simulink model "three_tank_linearization"  (R2020b)
settings: Solver=ode15s  StartTime=0.0  StopTime=2000  FixedStep=1  RelTol=1e-8  EnableMultiTasking=on
libraries: simulink x7, pid_lib x3
settings Model: Creator=Karl  LastModifiedBy=Fuzz4
settings SolverCC: AlgebraicLoopSolver=LineSearch  AutoInsertRateTranBlk=on
settings DataIOCC: SaveFormat=Array  ReturnWorkspaceOutputs=off  OutputOption=SpecifiedOutputTimes  OutputTimes=[0:2000]
settings OptimizationCC: LifeSpan=inf
settings DebuggingCC: AlgebraicLoopMsg=none  UnderspecifiedInitializationDetection=Classic  MergeDetectMultiDrivingBlocksExec=none  SFUnexpectedBacktrackingDiag=warning  SFNoUnconditionalDefaultTransitionDiag=warning  SFExecutionAtInitializationDiag=none  ArithmeticOperatorsInVariantConditions=warning
settings HardwareCC: ProdBitPerPointer=32  ProdBitPerSizeT=32  ProdBitPerPtrDiffT=32  ProdLargestAtomicFloat=None  ProdIntDivRoundTo=Undefined  ProdEndianess=Unspecified  ProdWordSize=32  ProdHWDeviceType=32-bit Generic
settings ModelReferenceCC: PropagateSignalLabelsOutOfModel=off
settings SFSimCC: SimUseLocalCustomCode=off  CustomCodeUndefinedFunction=UseInterfaceOnly
settings RTWCC: RTWUseLocalCustomCode=off
settings CodeAppCC: StateflowObjectComments=on
settings GRTTargetCC: TargetLangStandard=C89/C90 (ANSI)
settings ConfigComp: CovMetricSettings=dw  CovSaveCumulativeToWorkspaceVar=on  CovSaveSingleToWorkspaceVar=on  CovExternalEMLEnable=off

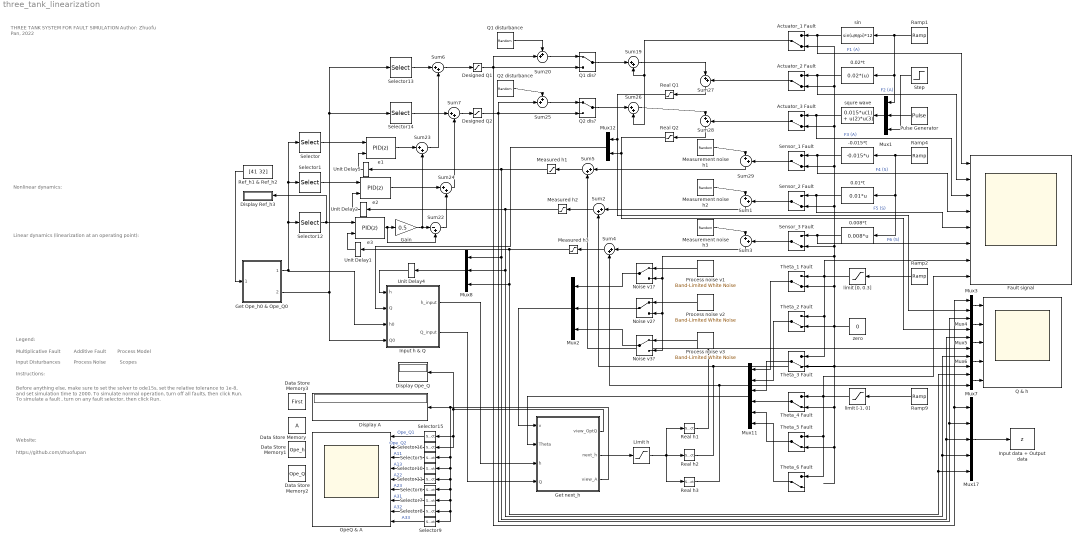
== system three_tank_linearization ==
  note: THREE TANK SYSTEM
      | FOR FAULT SIMULATION
      |
      | Author: Zhuofu Pan, 2022
  note: Multiplicative Fault
  note: Process Noise
  note: Process Model
  note: Input Disturbances
  note: Scopes
  note: Nonlinear dynamics:
  note: Linear dynamics
      | (linearization at an operating point):
  note: Before anything else, make sure to set the solver to ode15s, set the relative tolerance to 1e-8, and set simulation time to 2000.
      |
      | To simulate normal operation, turn off all faults, then click Run.
      |
      | To simulate a fault , turn on any fault selector, then click Run.
  note: Legend:
  note: Instructions:
  note: Website:
  note: https://github.com/zhuofupan
  note: Additive Fault
  " zero" : Constant  Value=0
  -0.015*t : Fcn  Expr=-0.015*u
  0.008*t : Fcn  Expr=0.008*u
  0.01*t : Fcn  Expr=0.01*u
  0.02*t : Fcn  Expr=0.02*(u)
  Actuator_1 Fault : ManualSwitch  CurrentSetting=0
  Actuator_2 Fault : ManualSwitch  CurrentSetting=0
  Actuator_3 Fault : ManualSwitch  CurrentSetting=0
  Data Store Memory : DataStoreMemory  ReadBeforeWriteMsg=warning  WriteAfterWriteMsg=warning  WriteAfterReadMsg=warning  ShowAdditionalParam=off  OutDataTypeStr=double  Dimensions=[3,3]
  Data Store Memory1 : DataStoreMemory  DataStoreName=Ope_h  ReadBeforeWriteMsg=warning  WriteAfterWriteMsg=warning  WriteAfterReadMsg=warning  ShowAdditionalParam=off  OutMin=0  OutMax=62  OutDataTypeStr=double  Dimensions=3
  Data Store Memory2 : DataStoreMemory  DataStoreName=Ope_Q  ReadBeforeWriteMsg=warning  WriteAfterWriteMsg=warning  WriteAfterReadMsg=warning  ShowAdditionalParam=off  OutMin=0  OutMax=150  OutDataTypeStr=double  Dimensions=2
  Data Store Memory3 : DataStoreMemory  DataStoreName=First  ReadBeforeWriteMsg=warning  WriteAfterWriteMsg=warning  WriteAfterReadMsg=warning  InitialValue=true  ShowAdditionalParam=off  OutDataTypeStr=boolean  Dimensions=1
  Designed Q1 : Saturate  UpperLimit=150  LowerLimit=0
  Designed Q2 : Saturate  UpperLimit=150  LowerLimit=0
  Display A : Display
      settings: Decimation=2
  Display Ope_Q : Display
  Display Ref_h3 : Display
  Fault signal : Scope  NumInputPorts=8
  Gain : Gain  Gain=0.5
  Get Ope_h0 & Ope_Q0 : MATLAB Function  TreatAsAtomicUnit=on
  Get next_h : MATLAB Function  TreatAsAtomicUnit=on
  Input data + Output data : ToWorkspace  VariableName=z  SampleTime=-1
  Input h & Q : MATLAB Function  TreatAsAtomicUnit=on
      settings: RTWSystemCode=Nonreusable function
  Limit h : Saturate  UpperLimit=62  LowerLimit=0
  Measured h1 : Saturate  UpperLimit=62  LowerLimit=0
  Measured h2 : Saturate  UpperLimit=62  LowerLimit=0
  Measured h3 : Saturate  UpperLimit=62  LowerLimit=0
  Measurement noise h1 : RandomNumber  Variance=0.01  Seed=randi(100000)
  Measurement noise h2 : RandomNumber  Variance=0.01  Seed=randi(100000)
  Measurement noise h3 : RandomNumber  Variance=0.01  Seed=randi(100000)
  Mux1 : Mux  Inputs=3
  Mux11 : Mux  Inputs=6
  Mux{3..7,12} (6 alike) : Mux  Inputs=2
  Mux17 : Mux  Inputs=5
  Mux2 : Mux  Inputs=3
  Mux8 : Mux  Inputs=3
  Noise v1? : ManualSwitch
  Noise v2? : ManualSwitch
  Noise v3? : ManualSwitch
  OpeQ & A : Scope  NumInputPorts=9
  Process noise v1 : simulink/Sources/Band-Limited White Noise  Cov=[1e-4]  Ts=1  seed=randi(100000)
  Process noise v2 : simulink/Sources/Band-Limited White Noise  Cov=[1e-4]  Ts=1  seed=randi(100000)
  Process noise v3 : simulink/Sources/Band-Limited White Noise  Cov=[1e-4]  Ts=1  seed=randi(100000)
  Pulse Generator : DiscretePulseGenerator  PulseType=Time based  Amplitude=5  Period=120  PulseWidth=80
  Q & h : Scope  NumInputPorts=5
  Q1 dis? : ManualSwitch
  Q1 disturbance : RandomNumber  Variance=0.01  Seed=randi(100000)  SampleTime=15
  Q2 dis? : ManualSwitch
  Q2 disturbance : RandomNumber  Variance=0.01  Seed=randi(100000)  SampleTime=15
  Ramp1 : simulink/Sources/Ramp  slope=1  start=200  InitialOutput=0
  Ramp2 : simulink/Sources/Ramp  slope=0.00005  start=200  InitialOutput=0
  Ramp4 : simulink/Sources/Ramp  slope=1  start=200  InitialOutput=0
  Ramp9 : simulink/Sources/Ramp  slope=-0.001  start=200  InitialOutput=0
  Real Q1 : Saturate  UpperLimit=150  LowerLimit=0
  Real Q2 : Saturate  UpperLimit=150  LowerLimit=0
  Real h1 : Selector  InputPortWidth=3  IndexOptions=Index vector (dialog)  Indices=1  OutputSizes=1
  Real h2 : Selector  InputPortWidth=3  IndexOptions=Index vector (dialog)  Indices=2  OutputSizes=1
  Real h3 : Selector  InputPortWidth=3  IndexOptions=Index vector (dialog)  Indices=3  OutputSizes=1
  Ref_h1 & Ref_h2 : Constant  Value=[41 32]
  Selector : Selector  InputPortWidth=3  IndexOptions=Index vector (dialog)  Indices=1  OutputSizes=1
  Selector1 : Selector  InputPortWidth=3  IndexOptions=Index vector (dialog)  Indices=2  OutputSizes=1
  Selector10 : Selector  NumberOfDimensions=2  InputPortWidth=2  IndexOptions=Index vector (dialog),Index vector (dialog)  Indices=1,3  OutputSizes=1,1
  Selector11 : Selector  NumberOfDimensions=2  InputPortWidth=2  IndexOptions=Index vector (dialog),Index vector (dialog)  Indices=2,2  OutputSizes=1,1
  Selector12 : Selector  InputPortWidth=3  IndexOptions=Index vector (dialog)  Indices=3  OutputSizes=1
  Selector13 : Selector  InputPortWidth=2  IndexOptions=Index vector (dialog)  Indices=1  OutputSizes=1
  Selector14 : Selector  InputPortWidth=2  IndexOptions=Index vector (dialog)  Indices=2  OutputSizes=1
  Selector15 : Selector  InputPortWidth=2  IndexOptions=Index vector (dialog)  Indices=1  OutputSizes=1
  Selector16 : Selector  InputPortWidth=2  IndexOptions=Index vector (dialog)  Indices=2  OutputSizes=1
  Selector5 : Selector  NumberOfDimensions=2  InputPortWidth=2  IndexOptions=Index vector (dialog),Index vector (dialog)  Indices=1,1  OutputSizes=1,1
  Selector6 : Selector  NumberOfDimensions=2  InputPortWidth=2  IndexOptions=Index vector (dialog),Index vector (dialog)  Indices=2,3  OutputSizes=1,1
  Selector7 : Selector  NumberOfDimensions=2  InputPortWidth=2  IndexOptions=Index vector (dialog),Index vector (dialog)  Indices=3,1  OutputSizes=1,1
  Selector8 : Selector  NumberOfDimensions=2  InputPortWidth=2  IndexOptions=Index vector (dialog),Index vector (dialog)  Indices=3,2  OutputSizes=1,1
  Selector9 : Selector  NumberOfDimensions=2  InputPortWidth=2  IndexOptions=Index vector (dialog),Index vector (dialog)  Indices=3,3  OutputSizes=1,1
  Sensor_1 Fault : ManualSwitch  CurrentSetting=0
  Sensor_2 Fault : ManualSwitch  CurrentSetting=0
  Sensor_3 Fault : ManualSwitch  CurrentSetting=0
  Step : Step  Time=200  SampleTime=1
  Sum{1..7,19,23..24,26..29} (14 alike) : Sum  Inputs=|++
  Sum20 : Sum  Inputs=++|
  Sum22 : Sum  Inputs=|-+
  Sum25 : Sum  Inputs=++|
  Theta_1 Fault : ManualSwitch  CurrentSetting=0
  Theta_2 Fault : ManualSwitch  CurrentSetting=0
  Theta_3 Fault : ManualSwitch  CurrentSetting=0
  Theta_4 Fault : ManualSwitch  CurrentSetting=0
  Theta_5 Fault : ManualSwitch  CurrentSetting=0
  Theta_6 Fault : ManualSwitch  CurrentSetting=0
  Unit Delay{1..2,4..5} (4 alike) : UnitDelay  SampleTime=-1  HasFrameUpgradeWarning=on
  e1 : pid_lib/PID Controller (2DOF)  Controller=PID  Form=Parallel  TimeDomain=Discrete-time  UseExternalTs=off  SampleTime=-1  IntegratorMethod=Forward Euler  FilterMethod=Forward Euler  ControllerParametersSource=internal  P=0.02  I=0.02  D=0  UseFilter=on  N=100  b=1  c=1  TunerSelectOption=Transfer Function Based (PID Tuner App)  InitialConditionSource=internal  InitialConditionForIntegrator=0  InitialConditionForFilter=0  DifferentiatorICPrevScaledInput=0  ExternalReset=none  TrackingMode=off  Kt=1  LimitOutput=off  SatLimitsSource=internal  UpperSaturationLimit=inf  LowerSaturationLimit=-inf  LinearizeAsGain=on  AntiWindupMode=none  Kb=1  POutMin=[]  POutMax=[]  IOutMin=[]  IOutMax=[]  DOutMin=[]  DOutMax=[]  NOutMin=[]  NOutMax=[]  bOutMin=[]  bOutMax=[]  cOutMin=[]  cOutMax=[]  SumOutMin=[]  SumOutMax=[]  SaturationOutMin=[]  SaturationOutMax=[]  PParamMin=[]  PParamMax=[]  IParamMin=[]  IParamMax=[]  DParamMin=[]  DParamMax=[]  NParamMin=[]  NParamMax=[]  bParamMin=[]  bParamMax=[]  cParamMin=[]  cParamMax=[]  KbParamMin=[]  KbParamMax=[]  KtParamMin=[]  KtParamMax=[]  KbOutMin=[]  KbOutMax=[]  KtOutMin=[]  KtOutMax=[]  IntegratorOutMin=[]  IntegratorOutMax=[]  FilterOutMin=[]  FilterOutMax=[]  SumI1OutMin=[]  SumI1OutMax=[]  SumI2OutMin=[]  SumI2OutMax=[]  SumI3OutMin=[]  SumI3OutMax=[]  SumI4OutMin=[]  SumI4OutMax=[]  SumDOutMin=[]  SumDOutMax=[]  Sum1OutMin=[]  Sum1OutMax=[]  Sum2OutMin=[]  Sum2OutMax=[]  Sum3OutMin=[]  Sum3OutMax=[]  DifferentiatorOutMin=[]  DifferentiatorOutMax=[]  FilterDiffOutCoefMin=[]  FilterDiffOutCoefMax=[]  ReciprocalOutMin=[]  ReciprocalOutMax=[]  SumDenOutMin=[]  SumDenOutMax=[]  SumNumOutMin=[]  SumNumOutMax=[]  DivideOutMin=[]  DivideOutMax=[]  UdiffTsProdOutMin=[]  UdiffTsProdOutMax=[]  NTsProdOutMin=[]  NTsProdOutMax=[]  UintegralTsProdOutMin=[]  UintegralTsProdOutMax=[]  UngainTsProdOutMin=[]  UngainTsProdOutMax=[]  IntegratorContinuousStateAttributes=''  IntegratorStateMustResolveToSignalObject=off  IntegratorRTWStateStorageClass=Auto  FilterContinuousStateAttributes=''  FilterStateMustResolveToSignalObject=off  FilterRTWStateStorageClass=Auto  ParallelPVariant=InternalParameters  IdealPVariant=Disabled  IVariant=InternalParameters  DVariant=InternalParameters  bVariant=InternalParameters  cVariant=InternalParameters  IntegratorVariant=Discrete  SatVariant=Disabled  AWVariant=Passthrough  PCopyVariant=Disabled  TRVariant=Disabled  FdbkBlocksVariant=Forward  IdealPFdbkVariant=Disabled  SatFdbkVariant=Disabled  DerivativeFilterVariant=ForwardEulerFilter  NVariant=InternalParameters  NCopyVariant=Disabled  FilterICVariant=InternalICsFilter  IntegratorICVariant=InternalICs  ExternalResetVariant=Disabled  TRSumVariant=Passthrough  SumFdbkVariant=Disabled  SumVariant=Sum_PID  TsampFilterVariant=InternalTs  TsampNgainVariant=Passthrough  TsampIntegralVariant=Passthrough  ExternalSaturationOutDataTypeStr=Inherit: Same as second input
      settings: SourceProductBaseCode=SL
  e2 : pid_lib/PID Controller (2DOF)  Controller=PID  Form=Parallel  TimeDomain=Discrete-time  UseExternalTs=off  SampleTime=-1  IntegratorMethod=Forward Euler  FilterMethod=Forward Euler  ControllerParametersSource=internal  P=0.02  I=0.02  D=0  UseFilter=on  N=100  b=1  c=1  TunerSelectOption=Transfer Function Based (PID Tuner App)  InitialConditionSource=internal  InitialConditionForIntegrator=0  InitialConditionForFilter=0  DifferentiatorICPrevScaledInput=0  ExternalReset=none  TrackingMode=off  Kt=1  LimitOutput=off  SatLimitsSource=internal  UpperSaturationLimit=inf  LowerSaturationLimit=-inf  LinearizeAsGain=on  AntiWindupMode=none  Kb=1  POutMin=[]  POutMax=[]  IOutMin=[]  IOutMax=[]  DOutMin=[]  DOutMax=[]  NOutMin=[]  NOutMax=[]  bOutMin=[]  bOutMax=[]  cOutMin=[]  cOutMax=[]  SumOutMin=[]  SumOutMax=[]  SaturationOutMin=[]  SaturationOutMax=[]  PParamMin=[]  PParamMax=[]  IParamMin=[]  IParamMax=[]  DParamMin=[]  DParamMax=[]  NParamMin=[]  NParamMax=[]  bParamMin=[]  bParamMax=[]  cParamMin=[]  cParamMax=[]  KbParamMin=[]  KbParamMax=[]  KtParamMin=[]  KtParamMax=[]  KbOutMin=[]  KbOutMax=[]  KtOutMin=[]  KtOutMax=[]  IntegratorOutMin=[]  IntegratorOutMax=[]  FilterOutMin=[]  FilterOutMax=[]  SumI1OutMin=[]  SumI1OutMax=[]  SumI2OutMin=[]  SumI2OutMax=[]  SumI3OutMin=[]  SumI3OutMax=[]  SumI4OutMin=[]  SumI4OutMax=[]  SumDOutMin=[]  SumDOutMax=[]  Sum1OutMin=[]  Sum1OutMax=[]  Sum2OutMin=[]  Sum2OutMax=[]  Sum3OutMin=[]  Sum3OutMax=[]  DifferentiatorOutMin=[]  DifferentiatorOutMax=[]  FilterDiffOutCoefMin=[]  FilterDiffOutCoefMax=[]  ReciprocalOutMin=[]  ReciprocalOutMax=[]  SumDenOutMin=[]  SumDenOutMax=[]  SumNumOutMin=[]  SumNumOutMax=[]  DivideOutMin=[]  DivideOutMax=[]  UdiffTsProdOutMin=[]  UdiffTsProdOutMax=[]  NTsProdOutMin=[]  NTsProdOutMax=[]  UintegralTsProdOutMin=[]  UintegralTsProdOutMax=[]  UngainTsProdOutMin=[]  UngainTsProdOutMax=[]  IntegratorContinuousStateAttributes=''  IntegratorStateMustResolveToSignalObject=off  IntegratorRTWStateStorageClass=Auto  FilterContinuousStateAttributes=''  FilterStateMustResolveToSignalObject=off  FilterRTWStateStorageClass=Auto  ParallelPVariant=InternalParameters  IdealPVariant=Disabled  IVariant=InternalParameters  DVariant=InternalParameters  bVariant=InternalParameters  cVariant=InternalParameters  IntegratorVariant=Discrete  SatVariant=Disabled  AWVariant=Passthrough  PCopyVariant=Disabled  TRVariant=Disabled  FdbkBlocksVariant=Forward  IdealPFdbkVariant=Disabled  SatFdbkVariant=Disabled  DerivativeFilterVariant=ForwardEulerFilter  NVariant=InternalParameters  NCopyVariant=Disabled  FilterICVariant=InternalICsFilter  IntegratorICVariant=InternalICs  ExternalResetVariant=Disabled  TRSumVariant=Passthrough  SumFdbkVariant=Disabled  SumVariant=Sum_PID  TsampFilterVariant=InternalTs  TsampNgainVariant=Passthrough  TsampIntegralVariant=Passthrough  ExternalSaturationOutDataTypeStr=Inherit: Same as second input
      settings: SourceProductBaseCode=SL
  e3 : pid_lib/PID Controller (2DOF)  Controller=PID  Form=Parallel  TimeDomain=Discrete-time  UseExternalTs=off  SampleTime=-1  IntegratorMethod=Forward Euler  FilterMethod=Forward Euler  ControllerParametersSource=internal  P=0.02  I=0.02  D=0  UseFilter=on  N=100  b=1  c=1  TunerSelectOption=Transfer Function Based (PID Tuner App)  InitialConditionSource=internal  InitialConditionForIntegrator=0  InitialConditionForFilter=0  DifferentiatorICPrevScaledInput=0  ExternalReset=none  TrackingMode=off  Kt=1  LimitOutput=off  SatLimitsSource=internal  UpperSaturationLimit=inf  LowerSaturationLimit=-inf  LinearizeAsGain=on  AntiWindupMode=none  Kb=1  POutMin=[]  POutMax=[]  IOutMin=[]  IOutMax=[]  DOutMin=[]  DOutMax=[]  NOutMin=[]  NOutMax=[]  bOutMin=[]  bOutMax=[]  cOutMin=[]  cOutMax=[]  SumOutMin=[]  SumOutMax=[]  SaturationOutMin=[]  SaturationOutMax=[]  PParamMin=[]  PParamMax=[]  IParamMin=[]  IParamMax=[]  DParamMin=[]  DParamMax=[]  NParamMin=[]  NParamMax=[]  bParamMin=[]  bParamMax=[]  cParamMin=[]  cParamMax=[]  KbParamMin=[]  KbParamMax=[]  KtParamMin=[]  KtParamMax=[]  KbOutMin=[]  KbOutMax=[]  KtOutMin=[]  KtOutMax=[]  IntegratorOutMin=[]  IntegratorOutMax=[]  FilterOutMin=[]  FilterOutMax=[]  SumI1OutMin=[]  SumI1OutMax=[]  SumI2OutMin=[]  SumI2OutMax=[]  SumI3OutMin=[]  SumI3OutMax=[]  SumI4OutMin=[]  SumI4OutMax=[]  SumDOutMin=[]  SumDOutMax=[]  Sum1OutMin=[]  Sum1OutMax=[]  Sum2OutMin=[]  Sum2OutMax=[]  Sum3OutMin=[]  Sum3OutMax=[]  DifferentiatorOutMin=[]  DifferentiatorOutMax=[]  FilterDiffOutCoefMin=[]  FilterDiffOutCoefMax=[]  ReciprocalOutMin=[]  ReciprocalOutMax=[]  SumDenOutMin=[]  SumDenOutMax=[]  SumNumOutMin=[]  SumNumOutMax=[]  DivideOutMin=[]  DivideOutMax=[]  UdiffTsProdOutMin=[]  UdiffTsProdOutMax=[]  NTsProdOutMin=[]  NTsProdOutMax=[]  UintegralTsProdOutMin=[]  UintegralTsProdOutMax=[]  UngainTsProdOutMin=[]  UngainTsProdOutMax=[]  IntegratorContinuousStateAttributes=''  IntegratorStateMustResolveToSignalObject=off  IntegratorRTWStateStorageClass=Auto  FilterContinuousStateAttributes=''  FilterStateMustResolveToSignalObject=off  FilterRTWStateStorageClass=Auto  ParallelPVariant=InternalParameters  IdealPVariant=Disabled  IVariant=InternalParameters  DVariant=InternalParameters  bVariant=InternalParameters  cVariant=InternalParameters  IntegratorVariant=Discrete  SatVariant=Disabled  AWVariant=Passthrough  PCopyVariant=Disabled  TRVariant=Disabled  FdbkBlocksVariant=Forward  IdealPFdbkVariant=Disabled  SatFdbkVariant=Disabled  DerivativeFilterVariant=ForwardEulerFilter  NVariant=InternalParameters  NCopyVariant=Disabled  FilterICVariant=InternalICsFilter  IntegratorICVariant=InternalICs  ExternalResetVariant=Disabled  TRSumVariant=Passthrough  SumFdbkVariant=Disabled  SumVariant=Sum_PID  TsampFilterVariant=InternalTs  TsampNgainVariant=Passthrough  TsampIntegralVariant=Passthrough  ExternalSaturationOutDataTypeStr=Inherit: Same as second input
      settings: SourceProductBaseCode=SL
  "limit [-1, 0]" : Saturate  UpperLimit=0  LowerLimit=-1
  "limit [0, 0.3]" : Saturate  UpperLimit=0.3  LowerLimit=0
  sin : Fcn  Expr=sin(u/6/pi)*12
  squre wave : Fcn  Expr=0.015*u(1) + u(2)*u(3)
  wires:
  Q1 dis?/1 -> Sum19/1
  Sum28/1 -> Real Q2/1
  Ramp2/1 -> "limit [0, 0.3]"/1
  Process noise v2/1 -> Noise v2?/1
  Process noise v3/1 -> Noise v3?/1
  Process noise v1/1 -> Noise v1?/1
  Sum20/1 -> Q1 dis?/1
  Q1 disturbance/1 -> Sum20/1
  Ramp9/1 -> "limit [-1, 0]"/1
  e1/1 -> Sum23/1
  e3/1 -> Sum22/2, Gain/1
  Gain/1 -> Sum22/1, Sum23/2
  Sum22/1 -> Sum24/2
  e2/1 -> Sum24/1
  Designed Q1/1 -> Mux3/1, Mux17/1, Q1 dis?/2, Sum20/2
  Sum25/1 -> Q2 dis?/1
  Q2 disturbance/1 -> Sum25/1
  Designed Q2/1 -> Mux17/2, Mux4/1, Q2 dis?/2, Sum25/2
  Actuator_1 Fault/1 -> Sum26/2, Sum19/2
  Sum27/1 -> Real Q1/1
  Q2 dis?/1 -> Sum26/1
  Sum19/1 -> Sum27/1
  Actuator_2 Fault/1 -> Sum27/2
  Sum26/1 -> Sum28/1
  Actuator_3 Fault/1 -> Sum28/2
  Sensor_1 Fault/1 -> Sum29/2
  Measurement noise h2/1 -> Sum1/1
  Measurement noise h1/1 -> Sum29/1
  Mux17/1 -> Input data + Output data/1
  Measured h1/1 -> Mux17/3, Mux5/1, Mux8/1, Unit Delay5/1
  Ramp1/1 -> Mux1/1, 0.02*t/1, sin/1
  Sum6/1 -> Designed Q1/1
  Sum7/1 -> Designed Q2/1
  Sensor_2 Fault/1 -> Sum1/2
  Measured h2/1 -> Mux17/4, Mux6/1, Mux8/2, Unit Delay2/1
  Sum1/1 -> Sum2/1
  Sensor_3 Fault/1 -> Sum3/2
  Measurement noise h3/1 -> Sum3/1
  Sum4/1 -> Measured h3/1
  Measured h3/1 -> Mux17/5, Mux7/1, Mux8/3, Unit Delay1/1
  Sum3/1 -> Sum4/1
  "limit [0, 0.3]"/1 -> Fault signal/7, Theta_1 Fault/1, Theta_3 Fault/1, Theta_2 Fault/1
  "limit [-1, 0]"/1 -> Theta_4 Fault/1, Fault signal/8, Theta_6 Fault/1, Theta_5 Fault/1
  sin/1 -> Fault signal/1, Actuator_1 Fault/1  "F1 (A)"
  0.02*t/1 -> Actuator_2 Fault/1, Fault signal/2  "F2 (A)"
  squre wave/1 -> Fault signal/3, Actuator_3 Fault/1  "F3 (A)"
  -0.015*t/1 -> Sensor_1 Fault/1, Fault signal/4  "F4 (S)"
  0.01*t/1 -> Fault signal/5, Sensor_2 Fault/1  "F5 (S)"
  0.008*t/1 -> Fault signal/6, Sensor_3 Fault/1  "F6 (S)"
  " zero"/1 -> Noise v1?/2, Noise v2?/2, Noise v3?/2, Actuator_1 Fault/2, Actuator_2 Fault/2, Actuator_3 Fault/2, Sensor_1 Fault/2, Sensor_2 Fault/2, Sensor_3 Fault/2, Theta_1 Fault/2, Theta_5 Fault/2, Theta_4 Fault/2, Theta_3 Fault/2, Theta_2 Fault/2
  Mux1/1 -> squre wave/1
  Pulse Generator/1 -> Mux1/2
  Step/1 -> Mux1/3
  Selector/1 -> e1/1
  Sum29/1 -> Sum5/1
  Noise v2?/1 -> Mux2/2
  Noise v1?/1 -> Mux2/1
  Noise v3?/1 -> Mux2/3
  Mux2/1 -> Get next_h/1(v)
  Theta_1 Fault/1 -> Mux11/1
  Theta_2 Fault/1 -> Mux11/2
  Theta_3 Fault/1 -> Mux11/3
  Theta_4 Fault/1 -> Mux11/4
  Theta_5 Fault/1 -> Mux11/5
  Theta_6 Fault/1 -> Mux11/6
  Real Q1/1 -> Mux3/2, Mux12/1
  Real Q2/1 -> Mux4/2, Mux12/2
  Sum23/1 -> Sum6/2
  Sum24/1 -> Sum7/2
  Mux3/1 -> Q & h/1
  Mux4/1 -> Q & h/2
  Mux5/1 -> Q & h/3
  Mux6/1 -> Q & h/4
  Mux7/1 -> Q & h/5
  Selector5/1 -> OpeQ & A/3  "A11"
  Selector10/1 -> OpeQ & A/4  "A13"
  Selector11/1 -> OpeQ & A/5  "A22"
  Selector6/1 -> OpeQ & A/6  "A23"
  Selector7/1 -> OpeQ & A/7  "A31"
  Selector8/1 -> OpeQ & A/8  "A32"
  Selector9/1 -> OpeQ & A/9  "A33"
  Get Ope_h0 & Ope_Q0/1(Ope_h0) -> Input h & Q/3(h0), Selector12/1, Selector1/1, Selector/1
  Mux11/1 -> Get next_h/2(Theta)
  Get next_h/3(view_A) -> Selector9/1, Selector8/1, Selector7/1, Selector6/1, Selector11/1, Selector10/1, Selector5/1, Display A/1
  Input h & Q/1(h_input) -> Get next_h/3(h)
  Input h & Q/2(Q_input) -> Get next_h/4(Q)
  Selector12/1 -> e3/1, Display Ref_h3/1
  Selector1/1 -> e2/1
  Mux12/1 -> Input h & Q/2(Q)
  Sum5/1 -> Measured h1/1
  Sum2/1 -> Measured h2/1
  Ramp4/1 -> -0.015*t/1, 0.01*t/1, 0.008*t/1
  Limit h/1 -> Real h3/1, Real h2/1, Real h1/1
  Real h1/1 -> Mux5/2, Sum5/2
  Real h2/1 -> Mux6/2, Sum2/2
  Real h3/1 -> Sum4/2, Mux7/2
  Get next_h/1(view_OptQ) -> Display Ope_Q/1, Selector16/1, Selector15/1
  Get next_h/2(next_h) -> Limit h/1
  Ref_h1 & Ref_h2/1 -> Get Ope_h0 & Ope_Q0/1(Ref_h12)
  Get Ope_h0 & Ope_Q0/2(Ope_Q0) -> Input h & Q/4(Q0), Selector14/1, Selector13/1
  Selector14/1 -> Sum7/1
  Selector13/1 -> Sum6/1
  Selector15/1 -> OpeQ & A/1  "Ope_Q1"
  Selector16/1 -> OpeQ & A/2  "Ope_Q2"
  Mux8/1 -> Unit Delay4/1
  Unit Delay4/1 -> Input h & Q/1(h)
  Unit Delay1/1 -> e3/2
  Unit Delay2/1 -> e2/2
  Unit Delay5/1 -> e1/2

== matlab function three_tank_linearization/Input h & Q ==
  settings: updateMethod=DISCRETE
  data: h_input output; h input; Q input; Q_input output; Ope_h data_store_memory; Ope_Q data_store_memory; h0 input; Q0 input; A data_store_memory; First data_store_memory
function [h_input, Q_input]= fcn(h, Q, h0, Q0)
    coder.extrinsic('Get_A');
    global A;
    global Ope_Q;
    global Ope_h;
    global First;
    
    if First
        First = false;
        h_input = h0;
        Q_input = Q0;
        Ope_h = h0;
        Ope_Q = Q0;
        Theta = [0, 0, 0, 0, 0, 0].';
        A = Get_A(Ope_h, Theta);
    else
        h_input = h;
        Q_input = Q;
    end
end

== matlab function three_tank_linearization/Get next_h ==
  settings: updateMethod=DISCRETE
  data: v input; Theta input; view_OptQ output; next_h output; h input; view_A output; Q input; A data_store_memory; Ope_h data_store_memory; Ope_Q data_store_memory
function [view_OptQ, next_h, view_A]= fcn(v, Theta, h, Q)
    coder.extrinsic('Get_A');
    coder.extrinsic('Get_OpeQ');
    coder.extrinsic('Solve_Opeh3');
    
    global A;
    global Ope_h;
    global Ope_Q;
    
    B = [1/154 0; 0 1/154; 0 0];
    next_h = A*(h - Ope_h) + B*(Q - Ope_Q) + v + Ope_h;
    
    % Get Ope_h3
    Ope_h = next_h;
    if Theta(3) == 0
        Ope_h(3) = ((0.46*(1+Theta(4)))^2 *Ope_h(1) + (0.45*(1+Theta(6)))^2 *Ope_h(2))/(0.46^2 + 0.45^2);
    else
        f = double(0);
        f = Solve_Opeh3(Ope_h(1), Ope_h(2), Ope_h(3), Theta(3), Theta(4), Theta(6));
        if f ~= 0
            % Find left_h3 & right_h3
            if f > 0
                % f(l_h3) >0
                l_h3 = Ope_h(3);
                r_h3 = l_h3;
                while f > 0 & r_h3 < 62
                    r_h3 = r_h3 + 1;
                    f = Solve_Opeh3(Ope_h(1), Ope_h(2), r_h3, Theta(3), Theta(4), Theta(6));
                end
                r_h3 = min(r_h3,62);
            else
                % f(r_h3) < 0
                r_h3 = Ope_h(3);
                l_h3 = r_h3;
                while f < 0 & l_h3 > 0
                    l_h3 = l_h3 - 1;
                    f = Solve_Opeh3(Ope_h(1), Ope_h(2), l_h3, Theta(3), Theta(4), Theta(6));
                end
                l_h3 = max(l_h3,0);
            end
            % Find middle_h3
            m_h3 = (l_h3 + r_h3)/2;
            cnt = 1;
            while abs(m_h3 - r_h3)>0.01 & abs(m_h3 - l_h3)>0.01 & cnt< 100
                f = Solve_Opeh3(Ope_h(1), Ope_h(2), m_h3, Theta(3), Theta(4), Theta(6));
                if f == 0
                    break;
                elseif f >0
                    l_h3 = m_h3;
                else
                    r_h3 = m_h3;
                end
                m_h3 = (l_h3 + r_h3)/2;
                cnt = cnt + 1;
            end
            Ope_h(3) = m_h3;
        end
    end
    Ope_h(Ope_h > 62) =62;
    Ope_h(Ope_h < 0) =0;
    
    % Get A & Ope_Q
    A = Get_A(Ope_h, Theta);
    Ope_Q = Get_OpeQ(A, Ope_h, Theta);
    
    view_A = A;
    view_OptQ = Ope_Q;
end

== matlab function three_tank_linearization/Get Ope_h0 & Ope_Q0 ==
  data: Ref_h12 input; Ope_h0 output; Ope_Q0 output
function [Ope_h0,Ope_Q0] = fcn(Ref_h12)
    coder.extrinsic('Get_A');
    coder.extrinsic('Get_OpeQ');
    A0 = zeros(3,3,'double');
    Ope_Q0 = zeros(2,1,'double');
    
    h1 = Ref_h12(1);
    h2 = Ref_h12(2);
    h3 = (0.46^2 *h1 + 0.45^2 *h2)/(0.46^2 + 0.45^2);
    Ope_h0 = [h1, h2, h3].';
    
    Theta = [0, 0, 0, 0, 0, 0].';
    A0 = Get_A(Ope_h0, Theta);
    Ope_Q0 = Get_OpeQ(A0, Ope_h0, Theta);
    
end
